simulink model "FIR_32tap_HIL"  (Simulink 7.0)
settings: Solver=FixedStepDiscrete  StartTime=0.0  StopTime=1024*sample_time  RelTol=1e-3
PreLoadFcn:
  | FIR_32tap_setup
InitFcn:
  | %% DSPBuilder Start
  | alt_dspbuilder_update_model(bdroot)
  | %% DSPBuilder End
values from neighbouring files (symbols this model uses):
  sample_time = 1/clock_freq    (= 1e-08)    [FIR_32tap_setup.m]
undefined symbols (not defined in the file or in its folder): get
libraries: allblocks_alteradspbuilder2 x9, dspsnks4 x2, simulink x1
settings Model: Creator=davlin  LastModifiedBy=davlin
settings DebuggingCC: SaveWithParameterizedLinksMsg=none
settings GRTTargetCC: TargetFcnLib=ansi_tfl_tmw.mat

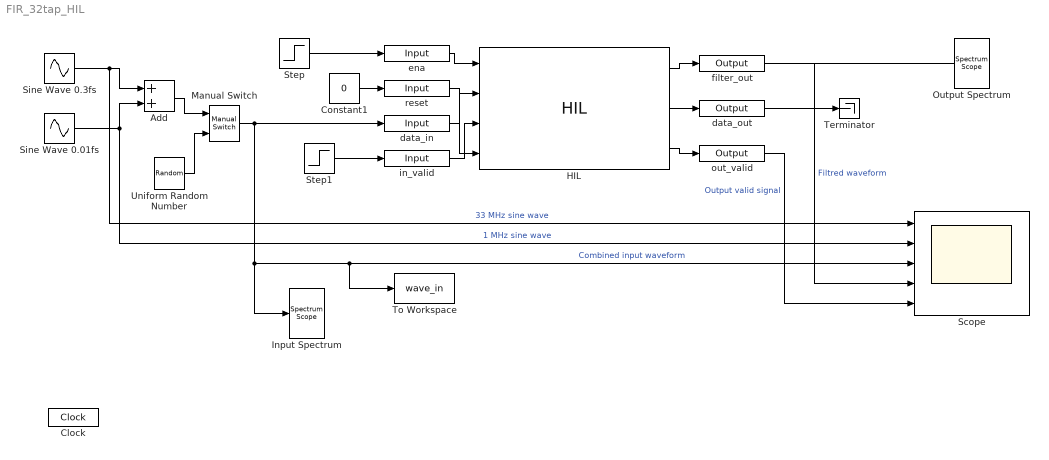
== system FIR_32tap_HIL ==
  Add : Sum  OutDataType=sfix(16)  OutScaling=2^-10
  Clock : allblocks_alteradspbuilder2/Clock  ClockPeriod=clock_period  ClockPeriodUnit=ns  SampleTime=sample_time  SimulationStartCycle=5  PhaseOffset=0  Reset=aclr  ResetType=Active Low  Export=off
  Constant1 : Constant  Value=0  OutDataType=sfix(16)  OutScaling=2^0  SampleTime=sample_time
  HIL : allblocks_alteradspbuilder2/HIL  entityName=FIR_32tap  inNames=ena data_in in_valid reset  inBwls="1  12   1   1   1   1"  inBwrs="0  0  0  0  0  0"  inTypes=b s b b  inDelayed="0  0  0  0"  outNames=filter_out data_out out_valid  outBwls="16  12   1"  outBwrs="11   0   0"  outTypes=f s b  resetNames=aclr  InputCount=6  InputNames=ena data_in Clock in_valid aclr reset  InputWidth="1  12   1   1   1   1"  InputRepresentation="0  1  0  0  0  0"  InputExport="0  0  2  0  3  0"  InputFPP="0  0  0  0  0  0"  OutputCount=3  OutputNames=filter_out data_out out_valid  OutputWidth="27  12   1"  OutputRepresentation="1  1  0"  OutputExport="0  0  0"  OutputFPP="11   0   0"  JtagCable=1  JtagDevice=1  BurstMode=off  BurstLength=1024  FrameMode=off  SOP=1  OutValid=1  QuartusProject=C:\Training\DSP_Training\Labs\DSPB_QII_V_9_0\sol\Ex3\partb\FIR_32tap_dspbuilder\FIR_32tap.qpf  HilNewConfig=off  ClockPinLocation=K17  ClockPinSource=0  HilDeviceOnBoard=EP2S60F1020C4ES  DR_length=48  dspbuilder_reset=on  SLD_NODE_INFO=6538956  AssertSclrBeforeSimulation=1  SampleTime=0  dspb_ver=0  ResetLevel=Active_High  JtagCableName=USB-Blaster [USB-0]  JtagDeviceName=@1: EP2S60ES (0x020930DD)  ClockNames=Clock
  Input Spectrum : dspsnks4/Spectrum Scope  DialogController=dspdialog.SpectrumScope  DialogControllerArgs=DataTag0  SystemSampleTime=-1  ScopeProperties=on  Domain=Frequency  HorizSpan=1  UseBuffer=on  BufferSize=128  Overlap=64  inpFftLenInherit=off  FFTlength=128  numAvg=2  DisplayProperties=off  AxisGrid=on  Memory=off  FrameNumber=on  AxisLegend=off  AxisZoom=off  OpenScopeAtSimStart=on  OpenScopeImmediately=off  FigPos=get(0,'defaultfigureposition')  AxisProperties=off  XUnits=Hertz  XRange=[0...Fs/2]  InheritXIncr=on  XIncr=1.0  XLabel=Samples  XLimit=Auto  YUnits=dB  XMax=1  XMin=0  YLabel=Magnitude-squared, dB  LineProperties=off  wintypeSpecScope=Kaiser  RsSpecScope=50  betaSpecScope=5  winsampSpecScope=Periodic
      settings: YMin=7.87541679161896  YMax=68.8425321075722
  Manual Switch : simulink/Signal Routing/Manual Switch  SystemSampleTime=-1  sw=1  action=0  varsize=off
  Output Spectrum : dspsnks4/Spectrum Scope  DialogController=dspdialog.SpectrumScope  DialogControllerArgs=DataTag1  SystemSampleTime=-1  ScopeProperties=on  Domain=Frequency  HorizSpan=1  UseBuffer=on  BufferSize=128  Overlap=64  inpFftLenInherit=off  FFTlength=128  numAvg=2  DisplayProperties=off  AxisGrid=on  Memory=off  FrameNumber=on  AxisLegend=off  AxisZoom=off  OpenScopeAtSimStart=on  OpenScopeImmediately=off  FigPos=get(0,'defaultfigureposition')  AxisProperties=off  XUnits=Hertz  XRange=[0...Fs/2]  InheritXIncr=on  XIncr=1.0  XLabel=Samples  XLimit=Auto  YUnits=dB  XMax=1  XMin=0  YLabel=Magnitude-squared, dB  LineProperties=off  wintypeSpecScope=Kaiser  RsSpecScope=50  betaSpecScope=5  winsampSpecScope=Periodic
      settings: YMin=-1.27620981719059  YMax=68.9549437099692
  Scope : Scope  NumInputPorts=5
      settings: YMin=-500~-750~-1000~-750~-5  YMax=500~750~1000~750~5  Decimation=sample_time  SampleInput=on  SampleTime=sample_time
  Sine Wave 0.01fs : Sin  SineType=Sample based  Amplitude=2^9-1  Samples=100  SampleTime=sample_time
  Sine Wave 0.3fs : Sin  SineType=Sample based  Amplitude=2^9-1  Samples=3  SampleTime=sample_time
  Step : Step  Time=sample_time  SampleTime=sample_time
  Step1 : Step  Time=sample_time  SampleTime=sample_time
  Terminator : Terminator
  To Workspace : ToWorkspace  VariableName=wave_in  SampleTime=-1  SaveFormat=Array
  Uniform Random Number : UniformRandomNumber  Minimum=-2^10  Maximum=2^10-1  SampleTime=sample_time
  data_in : allblocks_alteradspbuilder2/Input  iofile=C:\Training\DSP_Training\Labs\DSPB_QII_V_9_0\Sol\Ex3\partb\tb_FIR_32tap_HIL\FIR%5F32tap%5FHIL_data%5Fin.salt  BusType=Signed Integer  bwl=12  bwr=0  SpecifyClock=on  clock=Clock  PORTTYPE=Input  externalType=Inferred  allowFloatingPointOverride=on  logOutputs=off
  data_out : allblocks_alteradspbuilder2/Output  iofile=C:\Training\DSP_Training\Labs\DSPB_QII_V_9_0\Sol\Ex3\partb\tb_FIR_32tap_HIL\FIR%5F32tap%5FHIL_data%5Fout.capture  BusType=Signed Integer  bwl=12  bwr=0  externalType=Inferred  PORTTYPE=Output  allowFloatingPointOverride=on  logOutputs=off
  ena : allblocks_alteradspbuilder2/Input  iofile=C:\Training\DSP_Training\Labs\DSPB_QII_V_9_0\Sol\Ex3\partb\tb_FIR_32tap_HIL\FIR%5F32tap%5FHIL_ena.salt  BusType=Single Bit  bwl=8  bwr=0  SpecifyClock=on  clock=Clock  PORTTYPE=Input  externalType=Inferred  allowFloatingPointOverride=on  logOutputs=off
  filter_out : allblocks_alteradspbuilder2/Output  iofile=C:\Training\DSP_Training\Labs\DSPB_QII_V_9_0\Sol\Ex3\partb\tb_FIR_32tap_HIL\FIR%5F32tap%5FHIL_filter%5Fout.capture  BusType=Signed Fractional  bwl=16  bwr=11  externalType=Inferred  PORTTYPE=Output  allowFloatingPointOverride=on  logOutputs=off
  in_valid : allblocks_alteradspbuilder2/Input  iofile=C:\Training\DSP_Training\Labs\DSPB_QII_V_9_0\Sol\Ex3\partb\tb_FIR_32tap_HIL\FIR%5F32tap%5FHIL_in%5Fvalid.salt  BusType=Single Bit  bwl=8  bwr=0  SpecifyClock=on  clock=Clock  PORTTYPE=Input  externalType=Inferred  allowFloatingPointOverride=on  logOutputs=off
  out_valid : allblocks_alteradspbuilder2/Output  iofile=C:\Training\DSP_Training\Labs\DSPB_QII_V_9_0\Sol\Ex3\partb\tb_FIR_32tap_HIL\FIR%5F32tap%5FHIL_out%5Fvalid.capture  BusType=Single Bit  bwl=8  bwr=0  externalType=Inferred  PORTTYPE=Output  allowFloatingPointOverride=on  logOutputs=off
  reset : allblocks_alteradspbuilder2/Input  iofile=C:\Training\DSP_Training\Labs\DSPB_QII_V_9_0\Sol\Ex3\partb\tb_FIR_32tap_HIL\FIR%5F32tap%5FHIL_reset.salt  BusType=Single Bit  bwl=8  bwr=0  SpecifyClock=on  clock=Clock  PORTTYPE=Input  externalType=Inferred  allowFloatingPointOverride=on  logOutputs=off
  wires:
  Step/1 -> ena/1
  Constant1/1 -> reset/1
  Step1/1 -> in_valid/1
  filter_out/1 -> Output Spectrum/1, Scope/4  "Filtred waveform"
  Manual Switch/1 -> data_in/1, Input Spectrum/1, Scope/3, To Workspace/1  "Combined input waveform"
  Sine Wave 0.3fs/1 -> Add/1, Scope/1  "33 MHz sine wave"
  Sine Wave 0.01fs/1 -> Add/2, Scope/2  "1 MHz sine wave"
  Uniform Random Number/1 -> Manual Switch/2
  out_valid/1 -> Scope/5  "Output valid signal"
  Add/1 -> Manual Switch/1
  data_out/1 -> Terminator/1
  ena/1 -> HIL/1
  reset/1 -> HIL/4
  data_in/1 -> HIL/2
  in_valid/1 -> HIL/3
  HIL/1 -> filter_out/1
  HIL/2 -> data_out/1
  HIL/3 -> out_valid/1
